simulink model "mcs_1mch_70mhz2"  (R2013b)
settings: Solver=FixedStepDiscrete  SolverMode=SingleTasking  StartTime=0.0  StopTime=100000.0  FixedStep=0.1  RelTol=1e-3
undefined symbols (not defined in the file): xlfda_numerator, xlipgetpartsetting
libraries: xbsIndex_r4 x1766, xps_library x18, dspsigops x16, casper_library_misc x13, casper_library_delays x2, simulink x1
(part 3 of 18)

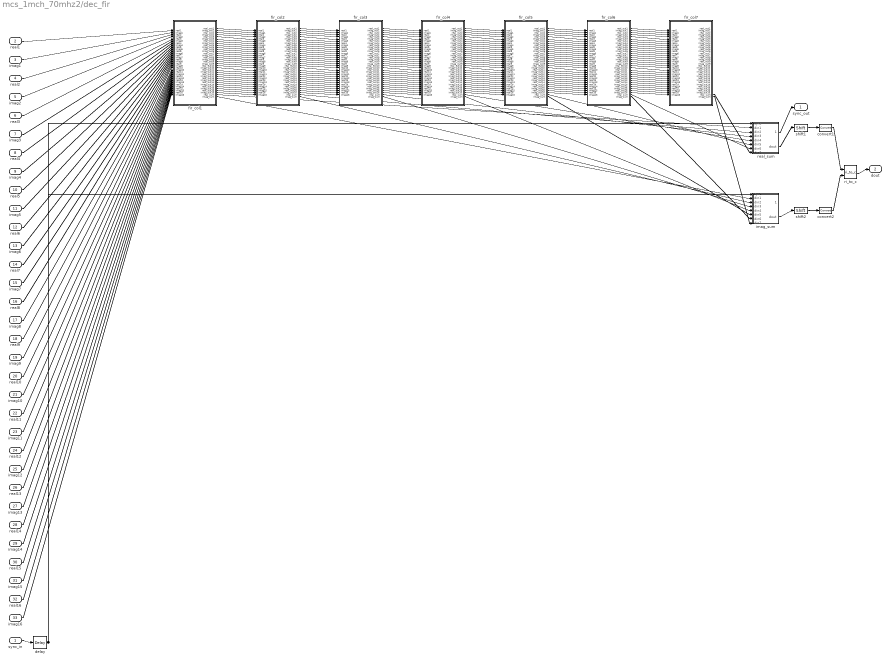
== system mcs_1mch_70mhz2/dec_fir ==
  sync_in : Inport
  real1 : Inport  Port=2
  imag1 : Inport  Port=3
  real2 : Inport  Port=4
  imag2 : Inport  Port=5
  real3 : Inport  Port=6
  imag3 : Inport  Port=7
  real4 : Inport  Port=8
  imag4 : Inport  Port=9
  real5 : Inport  Port=10
  imag5 : Inport  Port=11
  real6 : Inport  Port=12
  imag6 : Inport  Port=13
  real7 : Inport  Port=14
  imag7 : Inport  Port=15
  real8 : Inport  Port=16
  imag8 : Inport  Port=17
  real9 : Inport  Port=18
  imag9 : Inport  Port=19
  real10 : Inport  Port=20
  imag10 : Inport  Port=21
  real11 : Inport  Port=22
  imag11 : Inport  Port=23
  real12 : Inport  Port=24
  imag12 : Inport  Port=25
  real13 : Inport  Port=26
  imag13 : Inport  Port=27
  real14 : Inport  Port=28
  imag14 : Inport  Port=29
  real15 : Inport  Port=30
  imag15 : Inport  Port=31
  real16 : Inport  Port=32
  imag16 : Inport  Port=33
  convert1 : xbsIndex_r4/Convert  gui_display_data_type=Fixed-point  arith_type="Signed  (2's comp)"  n_bits=32  bin_pt=31  float_type=Single  exp_bits=8  fraction_bits=24  quantization="Round  (unbiased: +/- Inf)"  overflow=Wrap  en=off  latency=2  dbl_ovrd=off  pipeline=off  block_type=convert
  convert2 : xbsIndex_r4/Convert  gui_display_data_type=Fixed-point  arith_type="Signed  (2's comp)"  n_bits=32  bin_pt=31  float_type=Single  exp_bits=8  fraction_bits=24  quantization="Round  (unbiased: +/- Inf)"  overflow=Wrap  en=off  latency=2  dbl_ovrd=off  pipeline=off  block_type=convert
  delay : xbsIndex_r4/Delay  rst=off  infoeditControl=Selection of Reset will increase slice count due to use of real FFs and instead of SRLs  en=off  latency=8  dbl_ovrd=off  reg_retiming=off  block_type=delay
  fir_col1 : Subsystem  AncestorBlock=casper_library_downconverter/fir_col  mask(fir_col){n_inputs=16, coeff=[0.0075047   0.0067825   0.0058299   0.0046941   0.0034269   0.0020828  0.00071649 -0.00061865  -0.0018728  -0.0030011  -0.0039654  -0.0047353  -0.0052888   -0.005613  -0.0057043  -0.0055678], add_latency=1, mult_latency=2, coeff_bit_width=25, coeff_bin_pt=24, first_stage_hdl=on, adder_imp=DSP48}
      mask prompts: n_inputs "Inputs"; coeff "Coefficients"; add_latency "Add latency"; mult_latency "Mult Latency"; coeff_bit_width "Coefficient bit width"; coeff_bin_pt "Coefficient binary point"; first_stage_hdl "Implement first stage of adder trees on output as behavioural HDL"; adder_imp "Adder implementation"
      mask init:
      | fir_col_init(gcb, ...
      |     'n_inputs', n_inputs,...
      |     'coeff', coeff, ...
      |     'mult_latency', mult_latency, ...
      |     'add_latency', add_latency, ...
      |     'coeff_bit_width', coeff_bit_width, ...
      |     'coeff_bin_pt', coeff_bin_pt, ...
      |     'first_stage_hdl', first_stage_hdl, ...
      |     'adder_imp', adder_imp);
      mask Help: eval('xlWeb(''http://casper.berkeley.edu/wiki/Fir_col'')')
      mask TypeOptions adder_imp: Behavioral | Fabric | DSP48
  fir_col2 : Subsystem  AncestorBlock=casper_library_downconverter/fir_col  mask(fir_col){n_inputs=16, coeff=[-0.012687   -0.011457  -0.0098785  -0.0080348  -0.0060114  -0.0038941  -0.0017664  0.00029298   0.0022126   0.0039299   0.0053934   0.0065632   0.0074122   0.0079261   0.0081037   0.0079558], add_latency=1, mult_latency=2, coeff_bit_width=25, coeff_bin_pt=24, first_stage_hdl=on, adder_imp=DSP48}
      mask prompts: n_inputs "Inputs"; coeff "Coefficients"; add_latency "Add latency"; mult_latency "Mult Latency"; coeff_bit_width "Coefficient bit width"; coeff_bin_pt "Coefficient binary point"; first_stage_hdl "Implement first stage of adder trees on output as behavioural HDL"; adder_imp "Adder implementation"
      mask init: same as mcs_1mch_70mhz2/dec_fir/fir_col1
      mask Help: eval('xlWeb(''http://casper.berkeley.edu/wiki/Fir_col'')')
      mask TypeOptions adder_imp: Behavioral | Fabric | DSP48
  fir_col3 : Subsystem  AncestorBlock=casper_library_downconverter/fir_col  mask(fir_col){n_inputs=16, coeff=[0.037101    0.031646    0.026085    0.020538    0.015123   0.0099512   0.0051231  0.00072775  -0.0031605  -0.0064835  -0.0092001   -0.011287    -0.01274    -0.01357   -0.013806   -0.013493], add_latency=1, mult_latency=2, coeff_bit_width=25, coeff_bin_pt=24, first_stage_hdl=on, adder_imp=DSP48}
      mask prompts: n_inputs "Inputs"; coeff "Coefficients"; add_latency "Add latency"; mult_latency "Mult Latency"; coeff_bit_width "Coefficient bit width"; coeff_bin_pt "Coefficient binary point"; first_stage_hdl "Implement first stage of adder trees on output as behavioural HDL"; adder_imp "Adder implementation"
      mask init: same as mcs_1mch_70mhz2/dec_fir/fir_col1
      mask Help: eval('xlWeb(''http://casper.berkeley.edu/wiki/Fir_col'')')
      mask TypeOptions adder_imp: Behavioral | Fabric | DSP48
  fir_col4 : Subsystem  AncestorBlock=casper_library_downconverter/fir_col  mask(fir_col){n_inputs=16, coeff=[0.042327    0.047206    0.051624    0.055479    0.058679    0.061149     0.06283     0.06368     0.06368     0.06283    0.061149    0.058679    0.055479    0.051624    0.047206    0.042327], add_latency=1, mult_latency=2, coeff_bit_width=25, coeff_bin_pt=24, first_stage_hdl=on, adder_imp=DSP48}
      mask prompts: n_inputs "Inputs"; coeff "Coefficients"; add_latency "Add latency"; mult_latency "Mult Latency"; coeff_bit_width "Coefficient bit width"; coeff_bin_pt "Coefficient binary point"; first_stage_hdl "Implement first stage of adder trees on output as behavioural HDL"; adder_imp "Adder implementation"
      mask init: same as mcs_1mch_70mhz2/dec_fir/fir_col1
      mask Help: eval('xlWeb(''http://casper.berkeley.edu/wiki/Fir_col'')')
      mask TypeOptions adder_imp: Behavioral | Fabric | DSP48
  fir_col5 : Subsystem  AncestorBlock=casper_library_downconverter/fir_col  mask(fir_col){n_inputs=16, coeff=[-0.013493   -0.013806    -0.01357    -0.01274   -0.011287  -0.0092001  -0.0064835  -0.0031605  0.00072775   0.0051231   0.0099512    0.015123    0.020538    0.026085    0.031646    0.037101], add_latency=1, mult_latency=2, coeff_bit_width=25, coeff_bin_pt=24, first_stage_hdl=on, adder_imp=DSP48}
      mask prompts: n_inputs "Inputs"; coeff "Coefficients"; add_latency "Add latency"; mult_latency "Mult Latency"; coeff_bit_width "Coefficient bit width"; coeff_bin_pt "Coefficient binary point"; first_stage_hdl "Implement first stage of adder trees on output as behavioural HDL"; adder_imp "Adder implementation"
      mask init: same as mcs_1mch_70mhz2/dec_fir/fir_col1
      mask Help: eval('xlWeb(''http://casper.berkeley.edu/wiki/Fir_col'')')
      mask TypeOptions adder_imp: Behavioral | Fabric | DSP48
  fir_col6 : Subsystem  AncestorBlock=casper_library_downconverter/fir_col  mask(fir_col){n_inputs=16, coeff=[0.0079558   0.0081037   0.0079261   0.0074122   0.0065632   0.0053934   0.0039299   0.0022126  0.00029298  -0.0017664  -0.0038941  -0.0060114  -0.0080348  -0.0098785   -0.011457   -0.012687], add_latency=1, mult_latency=2, coeff_bit_width=25, coeff_bin_pt=24, first_stage_hdl=on, adder_imp=DSP48}
      mask prompts: n_inputs "Inputs"; coeff "Coefficients"; add_latency "Add latency"; mult_latency "Mult Latency"; coeff_bit_width "Coefficient bit width"; coeff_bin_pt "Coefficient binary point"; first_stage_hdl "Implement first stage of adder trees on output as behavioural HDL"; adder_imp "Adder implementation"
      mask init: same as mcs_1mch_70mhz2/dec_fir/fir_col1
      mask Help: eval('xlWeb(''http://casper.berkeley.edu/wiki/Fir_col'')')
      mask TypeOptions adder_imp: Behavioral | Fabric | DSP48
  fir_col7 : Subsystem  AncestorBlock=casper_library_downconverter/fir_col  mask(fir_col){n_inputs=16, coeff=[-0.0055678  -0.0057043   -0.005613  -0.0052888  -0.0047353  -0.0039654  -0.0030011  -0.0018728 -0.00061865  0.00071649   0.0020828   0.0034269   0.0046941   0.0058299   0.0067825   0.0075047], add_latency=1, mult_latency=2, coeff_bit_width=25, coeff_bin_pt=24, first_stage_hdl=on, adder_imp=DSP48}
      mask prompts: n_inputs "Inputs"; coeff "Coefficients"; add_latency "Add latency"; mult_latency "Mult Latency"; coeff_bit_width "Coefficient bit width"; coeff_bin_pt "Coefficient binary point"; first_stage_hdl "Implement first stage of adder trees on output as behavioural HDL"; adder_imp "Adder implementation"
      mask init: same as mcs_1mch_70mhz2/dec_fir/fir_col1
      mask Help: eval('xlWeb(''http://casper.berkeley.edu/wiki/Fir_col'')')
      mask TypeOptions adder_imp: Behavioral | Fabric | DSP48
  imag_sum : Subsystem  AncestorBlock=casper_library_misc/adder_tree  mask(adder_tree){n_inputs=7, latency=1, adder_imp=DSP48, first_stage_hdl=off}
      mask prompts: n_inputs "Number of Inputs"; latency "Add Latency"; adder_imp "Adder implementation"; first_stage_hdl "Use behavioural HDL for first stage of adders"
      mask help:
      | Sums all inputs using a tree of adds and delays.
      |
      | Number of inputs: The number of inputs to the block to be summed
      | Add latency: The number of clock cycles to perform one addition (affects timing)..
      | Adder implementation: choice of fabric or DSP48E core, or behavioral HDL
      | Use behavioural HDL for first stage of adders: Causes the first stage of adders to be absorbed into DSP blocks if multipliers precede them (Virtex 5). Overrides Adder implementation
      mask init:
      | adder_tree_init(gcb, ...
      |     'n_inputs', n_inputs, ...
      |     'latency', latency, ...
      |     'adder_imp', adder_imp, ...
      |     'first_stage_hdl', first_stage_hdl);
      settings: AttributesFormatString=latency 3
      mask Help: eval('xlWeb(''http://casper.berkeley.edu/wiki/Adder_tree'')')
      mask TypeOptions adder_imp: Behavioral | Fabric | DSP48
  real_sum : Subsystem  AncestorBlock=casper_library_misc/adder_tree  mask(adder_tree){n_inputs=7, latency=1, adder_imp=DSP48, first_stage_hdl=off}
      mask prompts: n_inputs "Number of Inputs"; latency "Add Latency"; adder_imp "Adder implementation"; first_stage_hdl "Use behavioural HDL for first stage of adders"
      mask help:
      | Sums all inputs using a tree of adds and delays.
      |
      | Number of inputs: The number of inputs to the block to be summed
      | Add latency: The number of clock cycles to perform one addition (affects timing)..
      | Adder implementation: choice of fabric or DSP48E core, or behavioral HDL
      | Use behavioural HDL for first stage of adders: Causes the first stage of adders to be absorbed into DSP blocks if multipliers precede them (Virtex 5). Overrides Adder implementation
      mask init:
      | adder_tree_init(gcb, ...
      |     'n_inputs', n_inputs, ...
      |     'latency', latency, ...
      |     'adder_imp', adder_imp, ...
      |     'first_stage_hdl', first_stage_hdl);
      settings: AttributesFormatString=latency 3
      mask Help: eval('xlWeb(''http://casper.berkeley.edu/wiki/Adder_tree'')')
      mask TypeOptions adder_imp: Behavioral | Fabric | DSP48
  ri_to_c : casper_library_misc/ri_to_c
  shift1 : xbsIndex_r4/Shift  shift_dir=Left  shift_bits=-8  en=off  latency=0  precision=Full  arith_type="Signed  (2's comp)"  n_bits=16  bin_pt=14  quantization=Truncate  overflow=Wrap  dbl_ovrd=off  block_type=shift
  shift2 : xbsIndex_r4/Shift  shift_dir=Left  shift_bits=-8  en=off  latency=0  precision=Full  arith_type="Signed  (2's comp)"  n_bits=16  bin_pt=14  quantization=Truncate  overflow=Wrap  dbl_ovrd=off  block_type=shift
  sync_out : Outport
  dout : Outport  Port=2
  wires:
  real1/1 -> fir_col1/1(real1)
  imag1/1 -> fir_col1/2(imag1)
  real2/1 -> fir_col1/3(real2)
  imag2/1 -> fir_col1/4(imag2)
  real3/1 -> fir_col1/5(real3)
  imag3/1 -> fir_col1/6(imag3)
  real4/1 -> fir_col1/7(real4)
  imag4/1 -> fir_col1/8(imag4)
  real5/1 -> fir_col1/9(real5)
  imag5/1 -> fir_col1/10(imag5)
  real6/1 -> fir_col1/11(real6)
  imag6/1 -> fir_col1/12(imag6)
  real7/1 -> fir_col1/13(real7)
  imag7/1 -> fir_col1/14(imag7)
  real8/1 -> fir_col1/15(real8)
  imag8/1 -> fir_col1/16(imag8)
  real9/1 -> fir_col1/17(real9)
  imag9/1 -> fir_col1/18(imag9)
  real10/1 -> fir_col1/19(real10)
  imag10/1 -> fir_col1/20(imag10)
  real11/1 -> fir_col1/21(real11)
  imag11/1 -> fir_col1/22(imag11)
  real12/1 -> fir_col1/23(real12)
  imag12/1 -> fir_col1/24(imag12)
  real13/1 -> fir_col1/25(real13)
  imag13/1 -> fir_col1/26(imag13)
  real14/1 -> fir_col1/27(real14)
  imag14/1 -> fir_col1/28(imag14)
  real15/1 -> fir_col1/29(real15)
  imag15/1 -> fir_col1/30(imag15)
  real16/1 -> fir_col1/31(real16)
  imag16/1 -> fir_col1/32(imag16)
  fir_col1/33(real_sum) -> real_sum/2(din1)
  fir_col1/34(imag_sum) -> imag_sum/2(din1)
  fir_col1/1(real_out1) -> fir_col2/1(real1)
  fir_col1/2(imag_out1) -> fir_col2/2(imag1)
  fir_col1/3(real_out2) -> fir_col2/3(real2)
  fir_col1/4(imag_out2) -> fir_col2/4(imag2)
  fir_col1/5(real_out3) -> fir_col2/5(real3)
  fir_col1/6(imag_out3) -> fir_col2/6(imag3)
  fir_col1/7(real_out4) -> fir_col2/7(real4)
  fir_col1/8(imag_out4) -> fir_col2/8(imag4)
  fir_col1/9(real_out5) -> fir_col2/9(real5)
  fir_col1/10(imag_out5) -> fir_col2/10(imag5)
  fir_col1/11(real_out6) -> fir_col2/11(real6)
  fir_col1/12(imag_out6) -> fir_col2/12(imag6)
  fir_col1/13(real_out7) -> fir_col2/13(real7)
  fir_col1/14(imag_out7) -> fir_col2/14(imag7)
  fir_col1/15(real_out8) -> fir_col2/15(real8)
  fir_col1/16(imag_out8) -> fir_col2/16(imag8)
  fir_col1/17(real_out9) -> fir_col2/17(real9)
  fir_col1/18(imag_out9) -> fir_col2/18(imag9)
  fir_col1/19(real_out10) -> fir_col2/19(real10)
  fir_col1/20(imag_out10) -> fir_col2/20(imag10)
  fir_col1/21(real_out11) -> fir_col2/21(real11)
  fir_col1/22(imag_out11) -> fir_col2/22(imag11)
  fir_col1/23(real_out12) -> fir_col2/23(real12)
  fir_col1/24(imag_out12) -> fir_col2/24(imag12)
  fir_col1/25(real_out13) -> fir_col2/25(real13)
  fir_col1/26(imag_out13) -> fir_col2/26(imag13)
  fir_col1/27(real_out14) -> fir_col2/27(real14)
  fir_col1/28(imag_out14) -> fir_col2/28(imag14)
  fir_col1/29(real_out15) -> fir_col2/29(real15)
  fir_col1/30(imag_out15) -> fir_col2/30(imag15)
  fir_col1/31(real_out16) -> fir_col2/31(real16)
  fir_col1/32(imag_out16) -> fir_col2/32(imag16)
  fir_col2/33(real_sum) -> real_sum/3(din2)
  fir_col2/34(imag_sum) -> imag_sum/3(din2)
  fir_col2/1(real_out1) -> fir_col3/1(real1)
  fir_col2/2(imag_out1) -> fir_col3/2(imag1)
  fir_col2/3(real_out2) -> fir_col3/3(real2)
  fir_col2/4(imag_out2) -> fir_col3/4(imag2)
  fir_col2/5(real_out3) -> fir_col3/5(real3)
  fir_col2/6(imag_out3) -> fir_col3/6(imag3)
  fir_col2/7(real_out4) -> fir_col3/7(real4)
  fir_col2/8(imag_out4) -> fir_col3/8(imag4)
  fir_col2/9(real_out5) -> fir_col3/9(real5)
  fir_col2/10(imag_out5) -> fir_col3/10(imag5)
  fir_col2/11(real_out6) -> fir_col3/11(real6)
  fir_col2/12(imag_out6) -> fir_col3/12(imag6)
  fir_col2/13(real_out7) -> fir_col3/13(real7)
  fir_col2/14(imag_out7) -> fir_col3/14(imag7)
  fir_col2/15(real_out8) -> fir_col3/15(real8)
  fir_col2/16(imag_out8) -> fir_col3/16(imag8)
  fir_col2/17(real_out9) -> fir_col3/17(real9)
  fir_col2/18(imag_out9) -> fir_col3/18(imag9)
  fir_col2/19(real_out10) -> fir_col3/19(real10)
  fir_col2/20(imag_out10) -> fir_col3/20(imag10)
  fir_col2/21(real_out11) -> fir_col3/21(real11)
  fir_col2/22(imag_out11) -> fir_col3/22(imag11)
  fir_col2/23(real_out12) -> fir_col3/23(real12)
  fir_col2/24(imag_out12) -> fir_col3/24(imag12)
  fir_col2/25(real_out13) -> fir_col3/25(real13)
  fir_col2/26(imag_out13) -> fir_col3/26(imag13)
  fir_col2/27(real_out14) -> fir_col3/27(real14)
  fir_col2/28(imag_out14) -> fir_col3/28(imag14)
  fir_col2/29(real_out15) -> fir_col3/29(real15)
  fir_col2/30(imag_out15) -> fir_col3/30(imag15)
  fir_col2/31(real_out16) -> fir_col3/31(real16)
  fir_col2/32(imag_out16) -> fir_col3/32(imag16)
  fir_col3/33(real_sum) -> real_sum/4(din3)
  fir_col3/34(imag_sum) -> imag_sum/4(din3)
  fir_col3/1(real_out1) -> fir_col4/1(real1)
  fir_col3/2(imag_out1) -> fir_col4/2(imag1)
  fir_col3/3(real_out2) -> fir_col4/3(real2)
  fir_col3/4(imag_out2) -> fir_col4/4(imag2)
  fir_col3/5(real_out3) -> fir_col4/5(real3)
  fir_col3/6(imag_out3) -> fir_col4/6(imag3)
  fir_col3/7(real_out4) -> fir_col4/7(real4)
  fir_col3/8(imag_out4) -> fir_col4/8(imag4)
  fir_col3/9(real_out5) -> fir_col4/9(real5)
  fir_col3/10(imag_out5) -> fir_col4/10(imag5)
  fir_col3/11(real_out6) -> fir_col4/11(real6)
  fir_col3/12(imag_out6) -> fir_col4/12(imag6)
  fir_col3/13(real_out7) -> fir_col4/13(real7)
  fir_col3/14(imag_out7) -> fir_col4/14(imag7)
  fir_col3/15(real_out8) -> fir_col4/15(real8)
  fir_col3/16(imag_out8) -> fir_col4/16(imag8)
  fir_col3/17(real_out9) -> fir_col4/17(real9)
  fir_col3/18(imag_out9) -> fir_col4/18(imag9)
  fir_col3/19(real_out10) -> fir_col4/19(real10)
  fir_col3/20(imag_out10) -> fir_col4/20(imag10)
  fir_col3/21(real_out11) -> fir_col4/21(real11)
  fir_col3/22(imag_out11) -> fir_col4/22(imag11)
  fir_col3/23(real_out12) -> fir_col4/23(real12)
  fir_col3/24(imag_out12) -> fir_col4/24(imag12)
  fir_col3/25(real_out13) -> fir_col4/25(real13)
  fir_col3/26(imag_out13) -> fir_col4/26(imag13)
  fir_col3/27(real_out14) -> fir_col4/27(real14)
  fir_col3/28(imag_out14) -> fir_col4/28(imag14)
  fir_col3/29(real_out15) -> fir_col4/29(real15)
  fir_col3/30(imag_out15) -> fir_col4/30(imag15)
  fir_col3/31(real_out16) -> fir_col4/31(real16)
  fir_col3/32(imag_out16) -> fir_col4/32(imag16)
  fir_col4/33(real_sum) -> real_sum/5(din4)
  fir_col4/34(imag_sum) -> imag_sum/5(din4)
  fir_col4/1(real_out1) -> fir_col5/1(real1)
  fir_col4/2(imag_out1) -> fir_col5/2(imag1)
  fir_col4/3(real_out2) -> fir_col5/3(real2)
  fir_col4/4(imag_out2) -> fir_col5/4(imag2)
  fir_col4/5(real_out3) -> fir_col5/5(real3)
  fir_col4/6(imag_out3) -> fir_col5/6(imag3)
  fir_col4/7(real_out4) -> fir_col5/7(real4)
  fir_col4/8(imag_out4) -> fir_col5/8(imag4)
  fir_col4/9(real_out5) -> fir_col5/9(real5)
  fir_col4/10(imag_out5) -> fir_col5/10(imag5)
  fir_col4/11(real_out6) -> fir_col5/11(real6)
  fir_col4/12(imag_out6) -> fir_col5/12(imag6)
  fir_col4/13(real_out7) -> fir_col5/13(real7)
  fir_col4/14(imag_out7) -> fir_col5/14(imag7)
  fir_col4/15(real_out8) -> fir_col5/15(real8)
  fir_col4/16(imag_out8) -> fir_col5/16(imag8)
  fir_col4/17(real_out9) -> fir_col5/17(real9)
  fir_col4/18(imag_out9) -> fir_col5/18(imag9)
  fir_col4/19(real_out10) -> fir_col5/19(real10)
  fir_col4/20(imag_out10) -> fir_col5/20(imag10)
  fir_col4/21(real_out11) -> fir_col5/21(real11)
  fir_col4/22(imag_out11) -> fir_col5/22(imag11)
  fir_col4/23(real_out12) -> fir_col5/23(real12)
  fir_col4/24(imag_out12) -> fir_col5/24(imag12)
  fir_col4/25(real_out13) -> fir_col5/25(real13)
  fir_col4/26(imag_out13) -> fir_col5/26(imag13)
  fir_col4/27(real_out14) -> fir_col5/27(real14)
  fir_col4/28(imag_out14) -> fir_col5/28(imag14)
  fir_col4/29(real_out15) -> fir_col5/29(real15)
  fir_col4/30(imag_out15) -> fir_col5/30(imag15)
  fir_col4/31(real_out16) -> fir_col5/31(real16)
  fir_col4/32(imag_out16) -> fir_col5/32(imag16)
  fir_col5/33(real_sum) -> real_sum/6(din5)
  fir_col5/34(imag_sum) -> imag_sum/6(din5)
  fir_col5/1(real_out1) -> fir_col6/1(real1)
  fir_col5/2(imag_out1) -> fir_col6/2(imag1)
  fir_col5/3(real_out2) -> fir_col6/3(real2)
  fir_col5/4(imag_out2) -> fir_col6/4(imag2)
  fir_col5/5(real_out3) -> fir_col6/5(real3)
  fir_col5/6(imag_out3) -> fir_col6/6(imag3)
  fir_col5/7(real_out4) -> fir_col6/7(real4)
  fir_col5/8(imag_out4) -> fir_col6/8(imag4)
  fir_col5/9(real_out5) -> fir_col6/9(real5)
  fir_col5/10(imag_out5) -> fir_col6/10(imag5)
  fir_col5/11(real_out6) -> fir_col6/11(real6)
  fir_col5/12(imag_out6) -> fir_col6/12(imag6)
  fir_col5/13(real_out7) -> fir_col6/13(real7)
  fir_col5/14(imag_out7) -> fir_col6/14(imag7)
  fir_col5/15(real_out8) -> fir_col6/15(real8)
  fir_col5/16(imag_out8) -> fir_col6/16(imag8)
  fir_col5/17(real_out9) -> fir_col6/17(real9)
  fir_col5/18(imag_out9) -> fir_col6/18(imag9)
  fir_col5/19(real_out10) -> fir_col6/19(real10)
  fir_col5/20(imag_out10) -> fir_col6/20(imag10)
  fir_col5/21(real_out11) -> fir_col6/21(real11)
  fir_col5/22(imag_out11) -> fir_col6/22(imag11)
  fir_col5/23(real_out12) -> fir_col6/23(real12)
  fir_col5/24(imag_out12) -> fir_col6/24(imag12)
  fir_col5/25(real_out13) -> fir_col6/25(real13)
  fir_col5/26(imag_out13) -> fir_col6/26(imag13)
  fir_col5/27(real_out14) -> fir_col6/27(real14)
  fir_col5/28(imag_out14) -> fir_col6/28(imag14)
  fir_col5/29(real_out15) -> fir_col6/29(real15)
  fir_col5/30(imag_out15) -> fir_col6/30(imag15)
  fir_col5/31(real_out16) -> fir_col6/31(real16)
  fir_col5/32(imag_out16) -> fir_col6/32(imag16)
  fir_col6/33(real_sum) -> real_sum/7(din6)
  fir_col6/34(imag_sum) -> imag_sum/7(din6)
  fir_col6/1(real_out1) -> fir_col7/1(real1)
  fir_col6/2(imag_out1) -> fir_col7/2(imag1)
  fir_col6/3(real_out2) -> fir_col7/3(real2)
  fir_col6/4(imag_out2) -> fir_col7/4(imag2)
  fir_col6/5(real_out3) -> fir_col7/5(real3)
  fir_col6/6(imag_out3) -> fir_col7/6(imag3)
  fir_col6/7(real_out4) -> fir_col7/7(real4)
  fir_col6/8(imag_out4) -> fir_col7/8(imag4)
  fir_col6/9(real_out5) -> fir_col7/9(real5)
  fir_col6/10(imag_out5) -> fir_col7/10(imag5)
  fir_col6/11(real_out6) -> fir_col7/11(real6)
  fir_col6/12(imag_out6) -> fir_col7/12(imag6)
  fir_col6/13(real_out7) -> fir_col7/13(real7)
  fir_col6/14(imag_out7) -> fir_col7/14(imag7)
  fir_col6/15(real_out8) -> fir_col7/15(real8)
  fir_col6/16(imag_out8) -> fir_col7/16(imag8)
  fir_col6/17(real_out9) -> fir_col7/17(real9)
  fir_col6/18(imag_out9) -> fir_col7/18(imag9)
  fir_col6/19(real_out10) -> fir_col7/19(real10)
  fir_col6/20(imag_out10) -> fir_col7/20(imag10)
  fir_col6/21(real_out11) -> fir_col7/21(real11)
  fir_col6/22(imag_out11) -> fir_col7/22(imag11)
  fir_col6/23(real_out12) -> fir_col7/23(real12)
  fir_col6/24(imag_out12) -> fir_col7/24(imag12)
  fir_col6/25(real_out13) -> fir_col7/25(real13)
  fir_col6/26(imag_out13) -> fir_col7/26(imag13)
  fir_col6/27(real_out14) -> fir_col7/27(real14)
  fir_col6/28(imag_out14) -> fir_col7/28(imag14)
  fir_col6/29(real_out15) -> fir_col7/29(real15)
  fir_col6/30(imag_out15) -> fir_col7/30(imag15)
  fir_col6/31(real_out16) -> fir_col7/31(real16)
  fir_col6/32(imag_out16) -> fir_col7/32(imag16)
  fir_col7/33(real_sum) -> real_sum/8(din7)
  fir_col7/34(imag_sum) -> imag_sum/8(din7)
  real_sum/2(dout) -> shift1/1
  imag_sum/2(dout) -> shift2/1
  shift1/1 -> convert1/1
  shift2/1 -> convert2/1
  convert1/1 -> ri_to_c/1
  convert2/1 -> ri_to_c/2
  ri_to_c/1 -> dout/1
  sync_in/1 -> delay/1
  delay/1 -> real_sum/1(sync), imag_sum/1(sync)
  real_sum/1(sync_out) -> sync_out/1

== system mcs_1mch_70mhz2/dout0_0 ==
  addr : Inport
  data_in : Inport  Port=2
  we : Inport  Port=3
  calc_add : Subsystem  mask{data_width=64, addr_width=9, sample_rate=sample_rate}
      mask prompts: data_width "data width"; addr_width "address width"; sample_rate "sample rate"
  convert_addr : xbsIndex_r4/Convert  gui_display_data_type=Fixed-point  arith_type=Unsigned  n_bits=addr_width  bin_pt=0  float_type=Single  exp_bits=8  fraction_bits=24  quantization=Truncate  overflow=Wrap  en=off  latency=0  dbl_ovrd=off  pipeline=off  block_type=convert
      settings: xl_area=[0, 0, 0, 0, 0, 0, 0]
  convert_din1 : xbsIndex_r4/Convert  gui_display_data_type=Fixed-point  arith_type=Unsigned  n_bits=64  bin_pt=0  float_type=Single  exp_bits=8  fraction_bits=24  quantization=Truncate  overflow=Wrap  en=off  latency=0  dbl_ovrd=off  pipeline=off  block_type=convert
      settings: xl_area=[0, 0, 0, 0, 0, 0, 0]
  convert_we : xbsIndex_r4/Convert  gui_display_data_type=Fixed-point  arith_type=Unsigned  n_bits=1  bin_pt=0  float_type=Single  exp_bits=8  fraction_bits=24  quantization=Truncate  overflow=Wrap  en=off  latency=0  dbl_ovrd=off  pipeline=off  block_type=convert
      settings: xl_area=[0, 0, 0, 0, 0, 0, 0]
  mcs_1mch_70mhz2_dout0_0_addr : xbsIndex_r4/Gateway Out  inherit_from_input=off  hdl_port=on  timing_constraint=None  locs_specified=off  LOCs={'A5','B9','A9','C1','A3','G6','E9','A6','A7','A8','B8','B1','B3','D9','B5','B4','B6','C2'}  UseAsDAC=off  DACChannel='1'  block_type=gatewayout
      settings: infoedit="Gateway out block.  Converts Xilinx fixed point inputs into ouputs of type Simulink integer, double, or fixed point.<P><P>Hardware notes:  In hardware these blocks become top level output ports or are discarded, depending on how they are configured."  xl_area=[0, 0, 0, 0, 0, 0, 0]  sginterface={'Nallatech'=>{'xdspkit'=>{'non_memory_mapped_port'=>'uprev_Shared_BRAM_addr'}},'Xilinx'=>{'jtaghwcosim'=>{'non_memory_mapped_port'=>'uprev_Shared_BRAM_addr'},'xdspkit'=>{'non_memory_mapped_port'=>'uprev_Shared_BRAM_addr'}}}
  mcs_1mch_70mhz2_dout0_0_data_in : xbsIndex_r4/Gateway Out  inherit_from_input=off  hdl_port=on  timing_constraint=None  locs_specified=off  LOCs={'B21','B22','A22','B23','B19','C19','A20','A21','A23','B24','A24','A25','E18','D18','C18','B18'}  UseAsDAC=off  DACChannel='1'  block_type=gatewayout
      settings: infoedit="Gateway out block.  Converts Xilinx fixed point inputs into ouputs of type Simulink integer, double, or fixed point.<P><P>Hardware notes:  In hardware these blocks become top level output ports or are discarded, depending on how they are configured."  xl_area=[0, 0, 0, 0, 0, 0, 0]  sginterface={'Nallatech'=>{'xdspkit'=>{'non_memory_mapped_port'=>'uprev_Shared_BRAM_data_in'}},'Xilinx'=>{'jtaghwcosim'=>{'non_memory_mapped_port'=>'uprev_Shared_BRAM_data_in'},'xdspkit'=>{'non_memory_mapped_port'=>'uprev_Shared_BRAM_data_in'}}}
  mcs_1mch_70mhz2_dout0_0_data_out : xbsIndex_r4/Gateway In  gui_display_data_type=Fixed-point  arith_type=Unsigned  n_bits=64  bin_pt=0  preci_type=Single  exp_width=8  frac_width=24  quantization=Truncate  overflow=Wrap  period=sample_rate  dbl_ovrd=off  timing_constraint=None  locs_specified=off  LOCs={}  UseAsADC=off  ADCChannel='1'  inherit_from_input=off  hdl_port=on  block_type=gatewayin
      settings: xl_area=[0, 0, 0, 0, 0, 0, 0]
  mcs_1mch_70mhz2_dout0_0_we : xbsIndex_r4/Gateway Out  inherit_from_input=off  hdl_port=on  timing_constraint=None  locs_specified=off  LOCs={'A14'}  UseAsDAC=off  DACChannel='1'  block_type=gatewayout
      settings: infoedit="Gateway out block.  Converts Xilinx fixed point inputs into ouputs of type Simulink integer, double, or fixed point.<P><P>Hardware notes:  In hardware these blocks become top level output ports or are discarded, depending on how they are configured."  xl_area=[0, 0, 0, 0, 0, 0, 0]
  mem : Subsystem
  munge_in : Subsystem  AncestorBlock=casper_library_flow_control/munge  mask(munge){divisions=2, div_size=[32 32], order=[1  0], arith_type_out=Unsigned, bin_pt_out=0}
      mask prompts: divisions "Number of divisions"; div_size "Division size (bits)"; order "Division packing order"; arith_type_out "Output arithmetic type"; bin_pt_out "Output binary point"
      mask help: Splits an input bus into the specified number of divisions and then recombines them in the order specified (most significant division = 0,least = number divisions-1)
      mask init:
      | munge_init(gcb, ...
      |     'divisions', divisions, ...
      |     'div_size', div_size, ...
      |     'order', order, ...
      |     'arith_type_out', arith_type_out, ...
      |     'bin_pt_out', bin_pt_out);
      settings: AttributesFormatString=|
      | split:[32 32]
      | join:[1 0]
      | Unsigned [64,0]
      mask TypeOptions arith_type_out: Unsigned | Signed  (2's comp) | Floating-point
  munge_out : Subsystem  AncestorBlock=casper_library_flow_control/munge  mask(munge){divisions=2, div_size=[32 32], order=[1  0], arith_type_out=Unsigned, bin_pt_out=0}
      mask prompts: divisions "Number of divisions"; div_size "Division size (bits)"; order "Division packing order"; arith_type_out "Output arithmetic type"; bin_pt_out "Output binary point"
      mask help: Splits an input bus into the specified number of divisions and then recombines them in the order specified (most significant division = 0,least = number divisions-1)
      mask init:
      | munge_init(gcb, ...
      |     'divisions', divisions, ...
      |     'div_size', div_size, ...
      |     'order', order, ...
      |     'arith_type_out', arith_type_out, ...
      |     'bin_pt_out', bin_pt_out);
      settings: AttributesFormatString=|
      | split:[32 32]
      | join:[1 0]
      | Unsigned [64,0]
      mask TypeOptions arith_type_out: Unsigned | Signed  (2's comp) | Floating-point
  data_out : Outport
  wires:
  convert_addr/1 -> mcs_1mch_70mhz2_dout0_0_addr/1
  convert_din1/1 -> mcs_1mch_70mhz2_dout0_0_data_in/1
  data_in/1 -> munge_in/1(din)
  calc_add/1(out) -> convert_addr/1
  mcs_1mch_70mhz2_dout0_0_we/1 -> mem/3(In3)
  mcs_1mch_70mhz2_dout0_0_data_in/1 -> mem/2(In2)
  mcs_1mch_70mhz2_dout0_0_addr/1 -> mem/1(In1)
  convert_we/1 -> mcs_1mch_70mhz2_dout0_0_we/1
  mcs_1mch_70mhz2_dout0_0_data_out/1 -> munge_out/1(din)
  mem/1(Out1) -> mcs_1mch_70mhz2_dout0_0_data_out/1
  addr/1 -> calc_add/1(in)
  we/1 -> convert_we/1
  munge_out/1(dout) -> data_out/1
  munge_in/1(dout) -> convert_din1/1

== system mcs_1mch_70mhz2/dout1_0 ==
  addr : Inport
  data_in : Inport  Port=2
  we : Inport  Port=3
  calc_add : Subsystem  mask{data_width=64, addr_width=9, sample_rate=sample_rate}
      mask prompts: data_width "data width"; addr_width "address width"; sample_rate "sample rate"
  convert_addr : xbsIndex_r4/Convert  gui_display_data_type=Fixed-point  arith_type=Unsigned  n_bits=addr_width  bin_pt=0  float_type=Single  exp_bits=8  fraction_bits=24  quantization=Truncate  overflow=Wrap  en=off  latency=0  dbl_ovrd=off  pipeline=off  block_type=convert
      settings: xl_area=[0, 0, 0, 0, 0, 0, 0]
  convert_din1 : xbsIndex_r4/Convert  gui_display_data_type=Fixed-point  arith_type=Unsigned  n_bits=64  bin_pt=0  float_type=Single  exp_bits=8  fraction_bits=24  quantization=Truncate  overflow=Wrap  en=off  latency=0  dbl_ovrd=off  pipeline=off  block_type=convert
      settings: xl_area=[0, 0, 0, 0, 0, 0, 0]
  convert_we : xbsIndex_r4/Convert  gui_display_data_type=Fixed-point  arith_type=Unsigned  n_bits=1  bin_pt=0  float_type=Single  exp_bits=8  fraction_bits=24  quantization=Truncate  overflow=Wrap  en=off  latency=0  dbl_ovrd=off  pipeline=off  block_type=convert
      settings: xl_area=[0, 0, 0, 0, 0, 0, 0]
  mcs_1mch_70mhz2_dout1_0_addr : xbsIndex_r4/Gateway Out  inherit_from_input=off  hdl_port=on  timing_constraint=None  locs_specified=off  LOCs={'A5','B9','A9','C1','A3','G6','E9','A6','A7','A8','B8','B1','B3','D9','B5','B4','B6','C2'}  UseAsDAC=off  DACChannel='1'  block_type=gatewayout
      settings: infoedit="Gateway out block.  Converts Xilinx fixed point inputs into ouputs of type Simulink integer, double, or fixed point.<P><P>Hardware notes:  In hardware these blocks become top level output ports or are discarded, depending on how they are configured."  xl_area=[0, 0, 0, 0, 0, 0, 0]  sginterface={'Nallatech'=>{'xdspkit'=>{'non_memory_mapped_port'=>'uprev_Shared_BRAM_addr'}},'Xilinx'=>{'jtaghwcosim'=>{'non_memory_mapped_port'=>'uprev_Shared_BRAM_addr'},'xdspkit'=>{'non_memory_mapped_port'=>'uprev_Shared_BRAM_addr'}}}
  mcs_1mch_70mhz2_dout1_0_data_in : xbsIndex_r4/Gateway Out  inherit_from_input=off  hdl_port=on  timing_constraint=None  locs_specified=off  LOCs={'B21','B22','A22','B23','B19','C19','A20','A21','A23','B24','A24','A25','E18','D18','C18','B18'}  UseAsDAC=off  DACChannel='1'  block_type=gatewayout
      settings: infoedit="Gateway out block.  Converts Xilinx fixed point inputs into ouputs of type Simulink integer, double, or fixed point.<P><P>Hardware notes:  In hardware these blocks become top level output ports or are discarded, depending on how they are configured."  xl_area=[0, 0, 0, 0, 0, 0, 0]  sginterface={'Nallatech'=>{'xdspkit'=>{'non_memory_mapped_port'=>'uprev_Shared_BRAM_data_in'}},'Xilinx'=>{'jtaghwcosim'=>{'non_memory_mapped_port'=>'uprev_Shared_BRAM_data_in'},'xdspkit'=>{'non_memory_mapped_port'=>'uprev_Shared_BRAM_data_in'}}}
  mcs_1mch_70mhz2_dout1_0_data_out : xbsIndex_r4/Gateway In  gui_display_data_type=Fixed-point  arith_type=Unsigned  n_bits=64  bin_pt=0  preci_type=Single  exp_width=8  frac_width=24  quantization=Truncate  overflow=Wrap  period=sample_rate  dbl_ovrd=off  timing_constraint=None  locs_specified=off  LOCs={}  UseAsADC=off  ADCChannel='1'  inherit_from_input=off  hdl_port=on  block_type=gatewayin
      settings: xl_area=[0, 0, 0, 0, 0, 0, 0]
  mcs_1mch_70mhz2_dout1_0_we : xbsIndex_r4/Gateway Out  inherit_from_input=off  hdl_port=on  timing_constraint=None  locs_specified=off  LOCs={'A14'}  UseAsDAC=off  DACChannel='1'  block_type=gatewayout
      settings: infoedit="Gateway out block.  Converts Xilinx fixed point inputs into ouputs of type Simulink integer, double, or fixed point.<P><P>Hardware notes:  In hardware these blocks become top level output ports or are discarded, depending on how they are configured."  xl_area=[0, 0, 0, 0, 0, 0, 0]
  mem : Subsystem
  munge_in : Subsystem  AncestorBlock=casper_library_flow_control/munge  mask(munge){divisions=2, div_size=[32 32], order=[1  0], arith_type_out=Unsigned, bin_pt_out=0}
      mask prompts: divisions "Number of divisions"; div_size "Division size (bits)"; order "Division packing order"; arith_type_out "Output arithmetic type"; bin_pt_out "Output binary point"
      mask help: Splits an input bus into the specified number of divisions and then recombines them in the order specified (most significant division = 0,least = number divisions-1)
      mask init:
      | munge_init(gcb, ...
      |     'divisions', divisions, ...
      |     'div_size', div_size, ...
      |     'order', order, ...
      |     'arith_type_out', arith_type_out, ...
      |     'bin_pt_out', bin_pt_out);
      settings: AttributesFormatString=|
      | split:[32 32]
      | join:[1 0]
      | Unsigned [64,0]
      mask TypeOptions arith_type_out: Unsigned | Signed  (2's comp) | Floating-point
  munge_out : Subsystem  AncestorBlock=casper_library_flow_control/munge  mask(munge){divisions=2, div_size=[32 32], order=[1  0], arith_type_out=Unsigned, bin_pt_out=0}
      mask prompts: divisions "Number of divisions"; div_size "Division size (bits)"; order "Division packing order"; arith_type_out "Output arithmetic type"; bin_pt_out "Output binary point"
      mask help: Splits an input bus into the specified number of divisions and then recombines them in the order specified (most significant division = 0,least = number divisions-1)
      mask init:
      | munge_init(gcb, ...
      |     'divisions', divisions, ...
      |     'div_size', div_size, ...
      |     'order', order, ...
      |     'arith_type_out', arith_type_out, ...
      |     'bin_pt_out', bin_pt_out);
      settings: AttributesFormatString=|
      | split:[32 32]
      | join:[1 0]
      | Unsigned [64,0]
      mask TypeOptions arith_type_out: Unsigned | Signed  (2's comp) | Floating-point
  data_out : Outport
  wires:
  munge_in/1(dout) -> convert_din1/1
  munge_out/1(dout) -> data_out/1
  we/1 -> convert_we/1
  addr/1 -> calc_add/1(in)
  mem/1(Out1) -> mcs_1mch_70mhz2_dout1_0_data_out/1
  mcs_1mch_70mhz2_dout1_0_data_out/1 -> munge_out/1(din)
  convert_we/1 -> mcs_1mch_70mhz2_dout1_0_we/1
  mcs_1mch_70mhz2_dout1_0_addr/1 -> mem/1(In1)
  mcs_1mch_70mhz2_dout1_0_data_in/1 -> mem/2(In2)
  mcs_1mch_70mhz2_dout1_0_we/1 -> mem/3(In3)
  calc_add/1(out) -> convert_addr/1
  data_in/1 -> munge_in/1(din)
  convert_din1/1 -> mcs_1mch_70mhz2_dout1_0_data_in/1
  convert_addr/1 -> mcs_1mch_70mhz2_dout1_0_addr/1

== system mcs_1mch_70mhz2/dout2_0 ==
  addr : Inport
  data_in : Inport  Port=2
  we : Inport  Port=3
  calc_add : Subsystem  mask{data_width=64, addr_width=16, sample_rate=sample_rate}
      mask prompts: data_width "data width"; addr_width "address width"; sample_rate "sample rate"
  convert_addr : xbsIndex_r4/Convert  gui_display_data_type=Fixed-point  arith_type=Unsigned  n_bits=addr_width  bin_pt=0  float_type=Single  exp_bits=8  fraction_bits=24  quantization=Truncate  overflow=Wrap  en=off  latency=0  dbl_ovrd=off  pipeline=off  block_type=convert
      settings: xl_area=[0, 0, 0, 0, 0, 0, 0]
  convert_din1 : xbsIndex_r4/Convert  gui_display_data_type=Fixed-point  arith_type=Unsigned  n_bits=64  bin_pt=0  float_type=Single  exp_bits=8  fraction_bits=24  quantization=Truncate  overflow=Wrap  en=off  latency=0  dbl_ovrd=off  pipeline=off  block_type=convert
      settings: xl_area=[0, 0, 0, 0, 0, 0, 0]
  convert_we : xbsIndex_r4/Convert  gui_display_data_type=Fixed-point  arith_type=Unsigned  n_bits=1  bin_pt=0  float_type=Single  exp_bits=8  fraction_bits=24  quantization=Truncate  overflow=Wrap  en=off  latency=0  dbl_ovrd=off  pipeline=off  block_type=convert
      settings: xl_area=[0, 0, 0, 0, 0, 0, 0]
  mcs_1mch_70mhz2_dout2_0_addr : xbsIndex_r4/Gateway Out  inherit_from_input=off  hdl_port=on  timing_constraint=None  locs_specified=off  LOCs={'A5','B9','A9','C1','A3','G6','E9','A6','A7','A8','B8','B1','B3','D9','B5','B4','B6','C2'}  UseAsDAC=off  DACChannel='1'  block_type=gatewayout
      settings: infoedit="Gateway out block.  Converts Xilinx fixed point inputs into ouputs of type Simulink integer, double, or fixed point.<P><P>Hardware notes:  In hardware these blocks become top level output ports or are discarded, depending on how they are configured."  xl_area=[0, 0, 0, 0, 0, 0, 0]  sginterface={'Nallatech'=>{'xdspkit'=>{'non_memory_mapped_port'=>'uprev_Shared_BRAM_addr'}},'Xilinx'=>{'jtaghwcosim'=>{'non_memory_mapped_port'=>'uprev_Shared_BRAM_addr'},'xdspkit'=>{'non_memory_mapped_port'=>'uprev_Shared_BRAM_addr'}}}
  mcs_1mch_70mhz2_dout2_0_data_in : xbsIndex_r4/Gateway Out  inherit_from_input=off  hdl_port=on  timing_constraint=None  locs_specified=off  LOCs={'B21','B22','A22','B23','B19','C19','A20','A21','A23','B24','A24','A25','E18','D18','C18','B18'}  UseAsDAC=off  DACChannel='1'  block_type=gatewayout
      settings: infoedit="Gateway out block.  Converts Xilinx fixed point inputs into ouputs of type Simulink integer, double, or fixed point.<P><P>Hardware notes:  In hardware these blocks become top level output ports or are discarded, depending on how they are configured."  xl_area=[0, 0, 0, 0, 0, 0, 0]  sginterface={'Nallatech'=>{'xdspkit'=>{'non_memory_mapped_port'=>'uprev_Shared_BRAM_data_in'}},'Xilinx'=>{'jtaghwcosim'=>{'non_memory_mapped_port'=>'uprev_Shared_BRAM_data_in'},'xdspkit'=>{'non_memory_mapped_port'=>'uprev_Shared_BRAM_data_in'}}}
  mcs_1mch_70mhz2_dout2_0_data_out : xbsIndex_r4/Gateway In  gui_display_data_type=Fixed-point  arith_type=Unsigned  n_bits=64  bin_pt=0  preci_type=Single  exp_width=8  frac_width=24  quantization=Truncate  overflow=Wrap  period=sample_rate  dbl_ovrd=off  timing_constraint=None  locs_specified=off  LOCs={}  UseAsADC=off  ADCChannel='1'  inherit_from_input=off  hdl_port=on  block_type=gatewayin
      settings: xl_area=[0, 0, 0, 0, 0, 0, 0]
  mcs_1mch_70mhz2_dout2_0_we : xbsIndex_r4/Gateway Out  inherit_from_input=off  hdl_port=on  timing_constraint=None  locs_specified=off  LOCs={'A14'}  UseAsDAC=off  DACChannel='1'  block_type=gatewayout
      settings: infoedit="Gateway out block.  Converts Xilinx fixed point inputs into ouputs of type Simulink integer, double, or fixed point.<P><P>Hardware notes:  In hardware these blocks become top level output ports or are discarded, depending on how they are configured."  xl_area=[0, 0, 0, 0, 0, 0, 0]
  mem : Subsystem
  munge_in : Subsystem  AncestorBlock=casper_library_flow_control/munge  mask(munge){divisions=2, div_size=[32 32], order=[1  0], arith_type_out=Unsigned, bin_pt_out=0}
      mask prompts: divisions "Number of divisions"; div_size "Division size (bits)"; order "Division packing order"; arith_type_out "Output arithmetic type"; bin_pt_out "Output binary point"
      mask help: Splits an input bus into the specified number of divisions and then recombines them in the order specified (most significant division = 0,least = number divisions-1)
      mask init:
      | munge_init(gcb, ...
      |     'divisions', divisions, ...
      |     'div_size', div_size, ...
      |     'order', order, ...
      |     'arith_type_out', arith_type_out, ...
      |     'bin_pt_out', bin_pt_out);
      settings: AttributesFormatString=|
      | split:[32 32]
      | join:[1 0]
      | Unsigned [64,0]
      mask TypeOptions arith_type_out: Unsigned | Signed  (2's comp) | Floating-point
  munge_out : Subsystem  AncestorBlock=casper_library_flow_control/munge  mask(munge){divisions=2, div_size=[32 32], order=[1  0], arith_type_out=Unsigned, bin_pt_out=0}
      mask prompts: divisions "Number of divisions"; div_size "Division size (bits)"; order "Division packing order"; arith_type_out "Output arithmetic type"; bin_pt_out "Output binary point"
      mask help: Splits an input bus into the specified number of divisions and then recombines them in the order specified (most significant division = 0,least = number divisions-1)
      mask init:
      | munge_init(gcb, ...
      |     'divisions', divisions, ...
      |     'div_size', div_size, ...
      |     'order', order, ...
      |     'arith_type_out', arith_type_out, ...
      |     'bin_pt_out', bin_pt_out);
      settings: AttributesFormatString=|
      | split:[32 32]
      | join:[1 0]
      | Unsigned [64,0]
      mask TypeOptions arith_type_out: Unsigned | Signed  (2's comp) | Floating-point
  data_out : Outport
  wires:
  munge_in/1(dout) -> convert_din1/1
  munge_out/1(dout) -> data_out/1
  we/1 -> convert_we/1
  addr/1 -> calc_add/1(in)
  mem/1(Out1) -> mcs_1mch_70mhz2_dout2_0_data_out/1
  mcs_1mch_70mhz2_dout2_0_data_out/1 -> munge_out/1(din)
  convert_we/1 -> mcs_1mch_70mhz2_dout2_0_we/1
  mcs_1mch_70mhz2_dout2_0_addr/1 -> mem/1(In1)
  mcs_1mch_70mhz2_dout2_0_data_in/1 -> mem/2(In2)
  mcs_1mch_70mhz2_dout2_0_we/1 -> mem/3(In3)
  calc_add/1(out) -> convert_addr/1
  data_in/1 -> munge_in/1(din)
  convert_din1/1 -> mcs_1mch_70mhz2_dout2_0_data_in/1
  convert_addr/1 -> mcs_1mch_70mhz2_dout2_0_addr/1

== system mcs_1mch_70mhz2/pipeline1 ==
  d : Inport
  Register0 : xbsIndex_r4/Register  init=0  rst=off  en=off  dbl_ovrd=off  block_type=register
      settings: block_version=11.4
  q : Outport
  wires:
  d/1 -> Register0/1
  Register0/1 -> q/1

== system mcs_1mch_70mhz2/pipeline10 ==
  d : Inport
  Register0 : xbsIndex_r4/Register  init=0  rst=off  en=off  dbl_ovrd=off  block_type=register
      settings: block_version=11.4
  q : Outport
  wires:
  d/1 -> Register0/1
  Register0/1 -> q/1

== system mcs_1mch_70mhz2/pipeline11 ==
  d : Inport
  Register0 : xbsIndex_r4/Register  init=0  rst=off  en=off  dbl_ovrd=off  block_type=register
      settings: block_version=11.4
  q : Outport
  wires:
  Register0/1 -> q/1
  d/1 -> Register0/1

== system mcs_1mch_70mhz2/pipeline110 ==
  d : Inport
  Register0 : xbsIndex_r4/Register  init=0  rst=off  en=off  dbl_ovrd=off  block_type=register
      settings: block_version=11.4
  Register1 : xbsIndex_r4/Register  init=0  rst=off  en=off  dbl_ovrd=off  block_type=register
  q : Outport
  wires:
  Register0/1 -> Register1/1
  d/1 -> Register0/1
  Register1/1 -> q/1

== system mcs_1mch_70mhz2/pipeline111 ==
  d : Inport
  Register0 : xbsIndex_r4/Register  init=0  rst=off  en=off  dbl_ovrd=off  block_type=register
      settings: block_version=11.4
  Register1 : xbsIndex_r4/Register  init=0  rst=off  en=off  dbl_ovrd=off  block_type=register
  q : Outport
  wires:
  Register0/1 -> Register1/1
  d/1 -> Register0/1
  Register1/1 -> q/1

== system mcs_1mch_70mhz2/pipeline112 ==
  d : Inport
  Register0 : xbsIndex_r4/Register  init=0  rst=off  en=off  dbl_ovrd=off  block_type=register
      settings: block_version=11.4
  Register1 : xbsIndex_r4/Register  init=0  rst=off  en=off  dbl_ovrd=off  block_type=register
  q : Outport
  wires:
  Register0/1 -> Register1/1
  d/1 -> Register0/1
  Register1/1 -> q/1

== system mcs_1mch_70mhz2/pipeline12 ==
  d : Inport
  Register0 : xbsIndex_r4/Register  init=0  rst=off  en=off  dbl_ovrd=off  block_type=register
      settings: block_version=11.4
  q : Outport
  wires:
  Register0/1 -> q/1
  d/1 -> Register0/1

== system mcs_1mch_70mhz2/pipeline13 ==
  d : Inport
  Register0 : xbsIndex_r4/Register  init=0  rst=off  en=off  dbl_ovrd=off  block_type=register
      settings: block_version=11.4
  q : Outport
  wires:
  d/1 -> Register0/1
  Register0/1 -> q/1

== system mcs_1mch_70mhz2/pipeline14 ==
  d : Inport
  Register0 : xbsIndex_r4/Register  init=0  rst=off  en=off  dbl_ovrd=off  block_type=register
      settings: block_version=11.4
  q : Outport
  wires:
  d/1 -> Register0/1
  Register0/1 -> q/1

== system mcs_1mch_70mhz2/pipeline143 ==
  d : Inport
  Register0 : xbsIndex_r4/Register  init=0  rst=off  en=off  dbl_ovrd=off  block_type=register
      settings: block_version=11.4
  Register1 : xbsIndex_r4/Register  init=0  rst=off  en=off  dbl_ovrd=off  block_type=register
      settings: block_version=11.4
  q : Outport
  wires:
  Register1/1 -> q/1
  d/1 -> Register0/1
  Register0/1 -> Register1/1

== system mcs_1mch_70mhz2/pipeline15 ==
  d : Inport
  Register0 : xbsIndex_r4/Register  init=0  rst=off  en=off  dbl_ovrd=off  block_type=register
      settings: block_version=11.4
  q : Outport
  wires:
  Register0/1 -> q/1
  d/1 -> Register0/1

== system mcs_1mch_70mhz2/pipeline16 ==
  d : Inport
  Register0 : xbsIndex_r4/Register  init=0  rst=off  en=off  dbl_ovrd=off  block_type=register
      settings: block_version=11.4
  q : Outport
  wires:
  d/1 -> Register0/1
  Register0/1 -> q/1

== system mcs_1mch_70mhz2/pipeline17 ==
  d : Inport
  Register0 : xbsIndex_r4/Register  init=0  rst=off  en=off  dbl_ovrd=off  block_type=register
      settings: block_version=11.4
  q : Outport
  wires:
  d/1 -> Register0/1
  Register0/1 -> q/1

== system mcs_1mch_70mhz2/pipeline18 ==
  d : Inport
  Register0 : xbsIndex_r4/Register  init=0  rst=off  en=off  dbl_ovrd=off  block_type=register
      settings: block_version=11.4
  q : Outport
  wires:
  Register0/1 -> q/1
  d/1 -> Register0/1

== system mcs_1mch_70mhz2/pipeline19 ==
  d : Inport
  Register0 : xbsIndex_r4/Register  init=0  rst=off  en=off  dbl_ovrd=off  block_type=register
      settings: block_version=11.4
  q : Outport
  wires:
  d/1 -> Register0/1
  Register0/1 -> q/1

== system mcs_1mch_70mhz2/pipeline2 ==
  d : Inport
  Register0 : xbsIndex_r4/Register  init=0  rst=off  en=off  dbl_ovrd=off  block_type=register
      settings: block_version=11.4
  q : Outport
  wires:
  Register0/1 -> q/1
  d/1 -> Register0/1

== system mcs_1mch_70mhz2/pipeline20 ==
  d : Inport
  Register0 : xbsIndex_r4/Register  init=0  rst=off  en=off  dbl_ovrd=off  block_type=register
      settings: block_version=11.4
  q : Outport
  wires:
  d/1 -> Register0/1
  Register0/1 -> q/1

== system mcs_1mch_70mhz2/pipeline21 ==
  d : Inport
  Register0 : xbsIndex_r4/Register  init=0  rst=off  en=off  dbl_ovrd=off  block_type=register
      settings: block_version=11.4
  Register1 : xbsIndex_r4/Register  init=0  rst=off  en=off  dbl_ovrd=off  block_type=register
      settings: block_version=11.4
  q : Outport
  wires:
  Register0/1 -> Register1/1
  d/1 -> Register0/1
  Register1/1 -> q/1

== system mcs_1mch_70mhz2/pipeline22 ==
  d : Inport
  Register0 : xbsIndex_r4/Register  init=0  rst=off  en=off  dbl_ovrd=off  block_type=register
      settings: block_version=11.4
  q : Outport
  wires:
  Register0/1 -> q/1
  d/1 -> Register0/1

== system mcs_1mch_70mhz2/pipeline23 ==
  d : Inport
  Register0 : xbsIndex_r4/Register  init=0  rst=off  en=off  dbl_ovrd=off  block_type=register
      settings: block_version=11.4
  q : Outport
  wires:
  Register0/1 -> q/1
  d/1 -> Register0/1

== system mcs_1mch_70mhz2/pipeline24 ==
  d : Inport
  Register0 : xbsIndex_r4/Register  init=0  rst=off  en=off  dbl_ovrd=off  block_type=register
      settings: block_version=11.4
  q : Outport
  wires:
  d/1 -> Register0/1
  Register0/1 -> q/1

== system mcs_1mch_70mhz2/pipeline25 ==
  d : Inport
  Register0 : xbsIndex_r4/Register  init=0  rst=off  en=off  dbl_ovrd=off  block_type=register
      settings: block_version=11.4
  q : Outport
  wires:
  d/1 -> Register0/1
  Register0/1 -> q/1

== system mcs_1mch_70mhz2/pipeline26 ==
  d : Inport
  Register0 : xbsIndex_r4/Register  init=0  rst=off  en=off  dbl_ovrd=off  block_type=register
      settings: block_version=11.4
  Register1 : xbsIndex_r4/Register  init=0  rst=off  en=off  dbl_ovrd=off  block_type=register
      settings: block_version=11.4
  q : Outport
  wires:
  Register1/1 -> q/1
  d/1 -> Register0/1
  Register0/1 -> Register1/1

== system mcs_1mch_70mhz2/pipeline27 ==
  d : Inport
  Register0 : xbsIndex_r4/Register  init=0  rst=off  en=off  dbl_ovrd=off  block_type=register
      settings: block_version=11.4
  Register1 : xbsIndex_r4/Register  init=0  rst=off  en=off  dbl_ovrd=off  block_type=register
      settings: block_version=11.4
  q : Outport
  wires:
  Register1/1 -> q/1
  d/1 -> Register0/1
  Register0/1 -> Register1/1

== system mcs_1mch_70mhz2/pipeline28 ==
  d : Inport
  Register0 : xbsIndex_r4/Register  init=0  rst=off  en=off  dbl_ovrd=off  block_type=register
      settings: block_version=11.4
  Register1 : xbsIndex_r4/Register  init=0  rst=off  en=off  dbl_ovrd=off  block_type=register
  q : Outport
  wires:
  Register0/1 -> Register1/1
  d/1 -> Register0/1
  Register1/1 -> q/1
